simulink model "speedctrl_virt_"  (Simulink 6.3)
settings: Solver=ode45  StartTime=0.0  StopTime=0.3  RelTol=1e-3
libraries: simulink_extras x1
settings Model: LastModifiedBy=jminor  StrictBusMsg=None
settings DataIOCC: MaxDataPoints=10000
settings OptimizationCC: BlockReduction=off  BooleanDataType=off
settings DebuggingCC: SolverPrmCheckMsg=none
settings HardwareCC: TargetUnknown=on

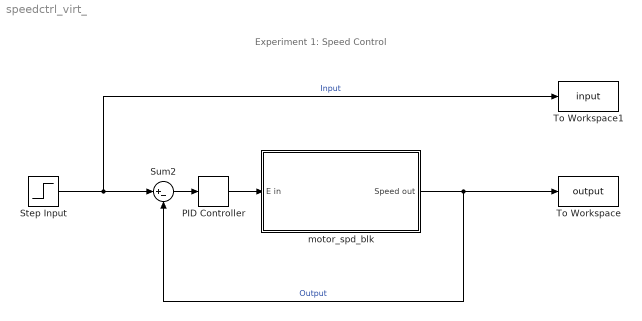
== system speedctrl_virt_ ==
  note: Experiment 1: Speed Control
  PID Controller : simulink_extras/Additional Linear/PID Controller  P=4  I=1.4  D=0
  Step Input : Step  Time=0  SampleTime=0
  Sum2 : Sum  Inputs=|+-  SaturateOnIntegerOverflow=on  InputSameDT=on
  To Workspace : ToWorkspace  VariableName=output  SampleTime=-1  SaveFormat=Structure With Time
  To Workspace1 : ToWorkspace  VariableName=input  SampleTime=-1  SaveFormat=Structure With Time
  motor_spd_blk : Subsystem
      mask Description: Real-Time Workshop generated S-function.
      mask Help: web(['file://',docroot,'/toolbox/rtw/rtwsfcn.html']);
      mask Display: disp('DC Motor (Speed Control)')
  wires:
  motor_spd_blk/1(Speed out) -> Sum2/2, To Workspace/1  "Output"
  PID Controller/1 -> motor_spd_blk/1(E in)
  Sum2/1 -> PID Controller/1
  Step Input/1 -> Sum2/1, To Workspace1/1  "Input"

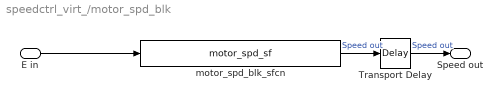
== system speedctrl_virt_/motor_spd_blk ==
  E in : Inport
  Transport Delay : TransportDelay  DelayTime=0.001
  motor_spd_blk_sfcn : S-Function  FunctionName=motor_spd_sf  SFunctionModules=""  mask{rtw_sf_name=motor_spd_sf, showVar=off}
      mask prompts: rtw_sf_name "Generated S-function name (model_sf):"; showVar "Show module list"
      mask help: Real-Time Workshop generated S-function.
      mask init:
      | displist = '';
      | if ~strcmp(get_param(gcb, 'FunctionName'), rtw_sf_name);
      |   set_param(gcb, 'FunctionName', rtw_sf_name);
      | end
      | if  showVar & exist('rtwsfunc') == 2
      |   tmplist = rtwsfunc(rtw_sf_name,gcb);
      |   tmplist = ['\nList of Modules:\n', tmplist];
      | elseif showVar
      |   tmplist = '\nList of Modules:\nRTW not licensed\n';
      | end
      | if showVar
      |   displist = tmplist;
      | end
      settings: CopyFcn=set_param(gcb,'linkstatus','none')
      mask Help: web(['file://',docroot,'/toolbox/rtw/rtwsfcn.html']);
      mask Display:
      | port_label('input',1,'E in');
      | port_label('output',1,'Speed out');
  Speed out : Outport
  wires:
  E in/1 -> motor_spd_blk_sfcn/1
  motor_spd_blk_sfcn/1 -> Transport Delay/1  "Speed out"
  Transport Delay/1 -> Speed out/1  "Speed out"
